simulink model "radar_subscription_brake"  (R2020a)
settings: Solver=VariableStepAuto  StartTime=0.0  StopTime=inf  RelTol=1e-3
undefined symbols (not defined in the file): Brake, Steer, Throttle
libraries: robotlib x3
settings Model: Creator=root  LastModifiedBy=root

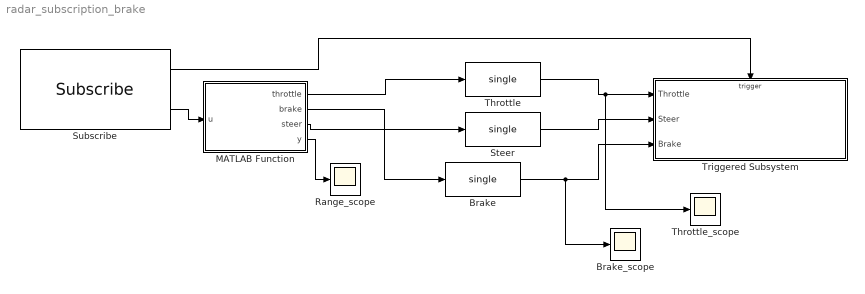
== system radar_subscription_brake ==
  Brake : DataTypeConversion  OutDataTypeStr=single
  Brake_scope : Scope
  MATLAB Function : MATLAB Function  TreatAsAtomicUnit=on
  Range_scope : Scope
  Steer : DataTypeConversion  OutDataTypeStr=single
  Subscribe : robotlib/Subscribe  topicSource=Select from ROS network  topic=/radar_processed_array  messageType=radar_msgs/RadarProcessedArray  sampleTime=-1  messageQueueLength=1
  Throttle : DataTypeConversion  OutDataTypeStr=single
  Throttle_scope : Scope
  Triggered Subsystem : Subsystem  TreatAsAtomicUnit=on
  wires:
  MATLAB Function/3(steer) -> Steer/1
  Subscribe/1 -> Triggered Subsystem/Trigger
  Subscribe/2 -> MATLAB Function/1(u)
  MATLAB Function/1(throttle) -> Throttle/1
  MATLAB Function/2(brake) -> Brake/1
  Throttle/1 -> Throttle_scope/1, Triggered Subsystem/1(Throttle)
  Steer/1 -> Triggered Subsystem/2(Steer)
  Brake/1 -> Brake_scope/1, Triggered Subsystem/3(Brake)
  MATLAB Function/4(y) -> Range_scope/1

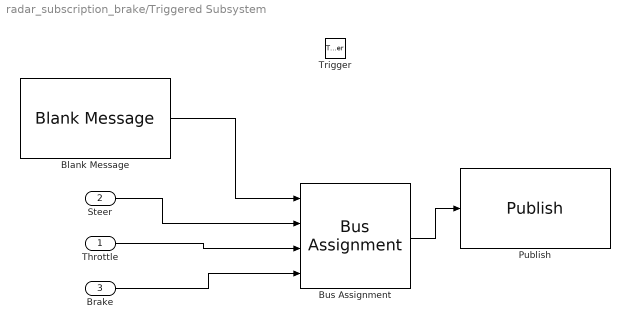
== system radar_subscription_brake/Triggered Subsystem ==
  Throttle : Inport
  Steer : Inport  Port=2
  Brake : Inport  Port=3
  Trigger : TriggerPort  VariantControl=Variant
  Blank Message : robotlib/Blank Message  messageClass=Message  entityType=ros_sut/ControlCommand  messageType=ros_sut/ControlCommand  SampleTime=inf
  Bus Assignment : BusAssignment  AssignedSignals=Steer,Throttle,Brake
  Publish : robotlib/Publish  topicSource=Select from ROS network  topic=/control_cmd  messageType=ros_sut/ControlCommand  messageQueueLength=1
  wires:
  Blank Message/1 -> Bus Assignment/1
  Bus Assignment/1 -> Publish/1
  Throttle/1 -> Bus Assignment/3
  Steer/1 -> Bus Assignment/2
  Brake/1 -> Bus Assignment/4

== matlab function radar_subscription_brake/MATLAB Function ==
  data: throttle output; brake output; u input; steer output; y output
function [throttle, brake, steer, y] = Range(u)
i = 1;
y = -10.0;


    while ( i < length(u.Groundtruth))
        range = u.Groundtruth(i,1).Range;
        object_type = u.Groundtruth(i,1).ObjectType;
        
        if (object_type == 2.0)
            y = range;
        end
        i = i + 1;
    end
    
    if y < 25
        steer = 0.0;
        brake = 100.0;
        throttle = 0.0;
    else
        steer = 0.0;
        brake = 0.0;
        throttle = 0.0;
    end
        

end
